simulink model "propulsion_system_simulation_with_solar_powered_battery"  (R2021a)
settings: Solver=VariableStepAuto  StartTime=0.0  StopTime=0.025  FixedStep=0.01  RelTol=1e-3
InitFcn:
  | prop_init_set
undefined symbols (not defined in the file or in its folder): Cp_total, Ct_total
libraries: spspowerguiLib x1
settings Model: SimulationMode=accelerator  Creator=76568  LastModifiedBy=76568

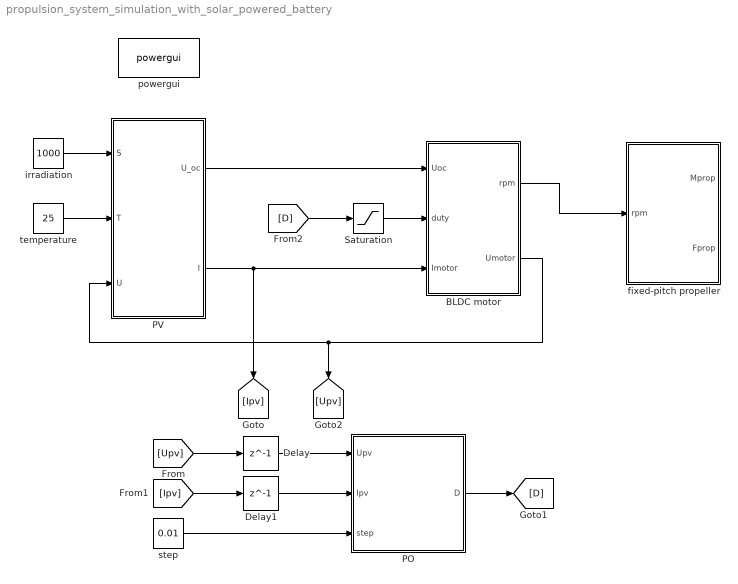
== system propulsion_system_simulation_with_solar_powered_battery ==
  BLDC motor : Subsystem  mask{Kv=125, Rm=0.184}
  Delay : Delay  DelayLength=1
  Delay1 : Delay  DelayLength=1
  PO : MATLAB Function  TreatAsAtomicUnit=on
  PV : Subsystem  mask{Uoc=31.464, Um=26.542, Isc=6.26, Im=5.87}
  Saturation : Saturate  UpperLimit=1  LowerLimit=0
  fixed-pitch propeller : Subsystem  mask{air_speed=10, prop_diameter=0.473, T_static=16.1936, T_max=6.85, V_max=15, air_rho=1.225}
  irradiation : Constant  Value=1000
  powergui : spspowerguiLib/powergui  Priority=1  SimulationMode=Continuous  SampleTime=0.01  frequency=60  Iterations=50  frequencyindice=0  Pbase=100e6  ErrMax=1e-4  UnitsV=kV  UnitsW=MW  buscounter=0  FunctionMessages=off  echomessages=off  EnableUseOfTLC=off  CurrentSourceSwitches=off  DisableSnubberDevices=off  DisableRonSwitches=off  DisableVfSwitches=off  DisplayEquations=off  AutomaticDiscreteSolvers=off  SolverType=Tustin/Backward Euler (TBE)  Interpol=off  ExternalGateDelay=off  methode=off  Ts=100  x0status=blocks  SPID=on  SwTol=0  HookPort=off  NonlinearTolerance=1e-4  nMaxIteration=100  ContinueOnMaxIteration=off  RestoreLinks=warning  ResistiveCurrentMeasurement=off  Frange=[0:2:500]  Ylog=off  Xlog=on  ShowGrid=off  save=off  variable=ZData  structure=0  ZoomFFT=off  StartTime=0.0  cycles=1  DisplayStyle=1  fundamental=60  FreqAxis=off  MaxFrequency=1000  frequencyindicesteady=1  RmsSteady=1  display=off
  step : Constant  Value=0.01
  temperature : Constant  Value=25
  wires:
  [Ipv] -> Delay1/1
  [Upv] -> Delay/1
  step/1 -> PO/3(step)
  PO/1(D) -> [D]
  irradiation/1 -> PV/1(S)
  temperature/1 -> PV/2(T)
  BLDC motor/1(rpm) -> fixed-pitch propeller/1(rpm)
  Saturation/1 -> BLDC motor/2(duty)
  Delay/1 -> PO/1(Upv)
  Delay1/1 -> PO/2(Ipv)
  [D] -> Saturation/1
  PV/1(U_oc) -> BLDC motor/1(Uoc)
  PV/2(I) -> [Ipv], BLDC motor/3(Imotor)
  BLDC motor/2(Umotor) -> [Upv], PV/3(U)

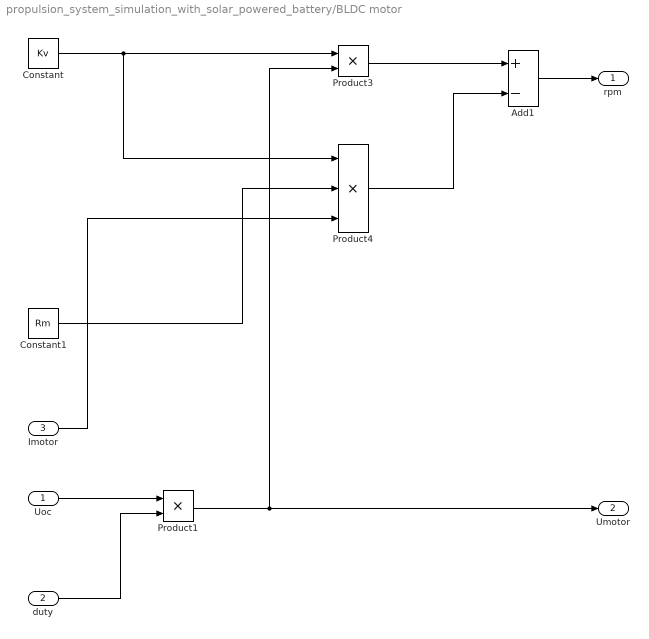
== system propulsion_system_simulation_with_solar_powered_battery/BLDC motor ==
  Uoc : Inport
  duty : Inport  Port=2
  Imotor : Inport  Port=3
  Add1 : Sum  Inputs=+-
  Constant : Constant  Value=Kv
  Constant1 : Constant  Value=Rm
  Product1 : Product
  Product3 : Product  Inputs=**
  Product4 : Product  Inputs=***
  rpm : Outport
  Umotor : Outport  Port=2
  wires:
  Constant/1 -> Product4/1, Product3/1
  Constant1/1 -> Product4/2
  Product3/1 -> Add1/1
  Product4/1 -> Add1/2
  duty/1 -> Product1/2
  Add1/1 -> rpm/1
  Imotor/1 -> Product4/3
  Uoc/1 -> Product1/1
  Product1/1 -> Umotor/1, Product3/2

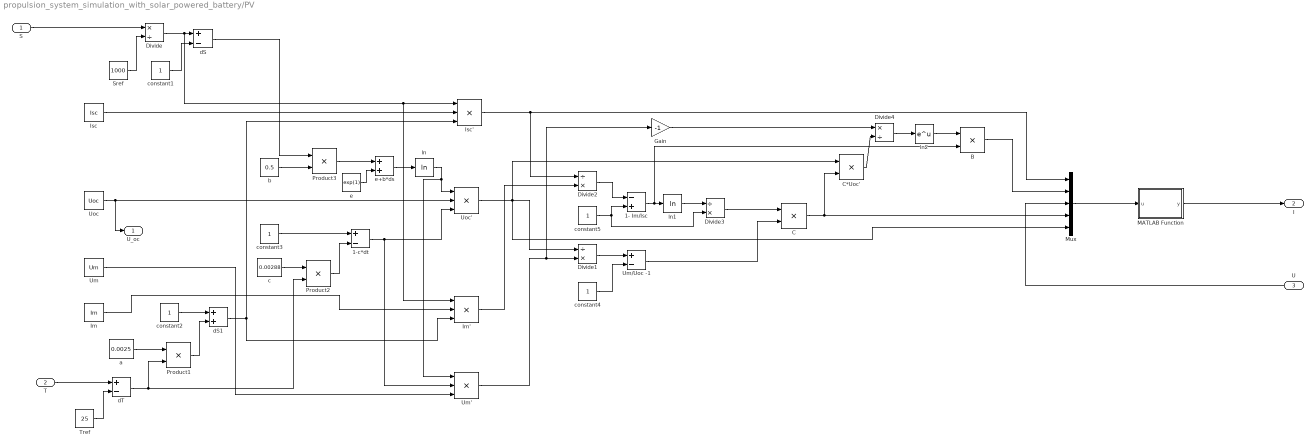
== system propulsion_system_simulation_with_solar_powered_battery/PV ==
  S : Inport
  T : Inport  Port=2
  U : Inport  Port=3
  1- Im/Isc : Sum  Inputs=-+
  1-c*dt : Sum  Inputs=+-
  B : Product
  C : Product
  C*Uoc' : Product
  Divide : Product  Inputs=*/
  Divide1 : Product  Inputs=/*
  Divide2 : Product  Inputs=/*
  Divide3 : Product  Inputs=/*
  Divide4 : Product  Inputs=*/
  Gain : Gain  Gain=-1
  Im : Constant  Value=Im
  Im' : Product  Inputs=3
  Isc : Constant  Value=Isc
  Isc' : Product  Inputs=3
  MATLAB Function : MATLAB Function  TreatAsAtomicUnit=on
  Mux : Mux  Inputs=5
  Product1 : Product
  Product2 : Product
  Product3 : Product
  Sref : Constant  Value=1000
  Tref : Constant  Value=25
  Um : Constant  Value=Um
  Um' : Product  Inputs=3
  Um/Uoc -1 : Sum  Inputs=+-
  Uoc : Constant  Value=Uoc
  Uoc' : Product  Inputs=3
  a : Constant  Value=0.0025
  b : Constant  Value=0.5
  c : Constant  Value=0.00288
  constant{1..5} (5 alike) : Constant
  dS : Sum  Inputs=+-
  dS1 : Sum
  dT : Sum  Inputs=+-
  e : Constant  Value=exp(1)
  e+b*ds : Sum
  ln : Math  Operator=log  SaturateOnIntegerOverflow=on
  ln1 : Math  Operator=log  SaturateOnIntegerOverflow=on
  ln2 : Math  SaturateOnIntegerOverflow=on
  U_oc : Outport
  I : Outport  Port=2
  wires:
  T/1 -> dT/1
  Tref/1 -> dT/2
  S/1 -> Divide/1
  Sref/1 -> Divide/2
  Divide/1 -> Isc'/1, Im'/1, dS/1
  constant1/1 -> dS/2
  a/1 -> Product1/1
  dT/1 -> Product2/2, Product1/2
  constant2/1 -> dS1/1
  Product1/1 -> dS1/2
  dS1/1 -> Im'/3, Isc'/3
  Isc/1 -> Isc'/2
  Uoc/1 -> U_oc/1, Uoc'/2
  constant3/1 -> 1-c*dt/1
  Product2/1 -> 1-c*dt/2
  c/1 -> Product2/1
  1-c*dt/1 -> Um'/2, Uoc'/3
  b/1 -> Product3/2
  dS/1 -> Product3/1
  e/1 -> e+b*ds/2
  Product3/1 -> e+b*ds/1
  e+b*ds/1 -> ln/1
  ln/1 -> Um'/1, Uoc'/1
  Im/1 -> Im'/2
  Um/1 -> Um'/3
  Um'/1 -> Gain/1, Divide1/2
  Divide1/1 -> Um/Uoc -1/1
  constant4/1 -> Um/Uoc -1/2
  Im'/1 -> Divide2/2
  Isc'/1 -> Mux/1, Divide2/1
  Divide2/1 -> 1- Im/Isc/1
  constant5/1 -> Divide3/2, 1- Im/Isc/2
  1- Im/Isc/1 -> B/2, ln1/1
  ln1/1 -> Divide3/1
  Um/Uoc -1/1 -> C/2
  Divide3/1 -> C/1
  C/1 -> Mux/4, C*Uoc'/2
  Gain/1 -> Divide4/1
  C*Uoc'/1 -> Divide4/2
  Divide4/1 -> ln2/1
  ln2/1 -> B/1
  B/1 -> Mux/2
  Uoc'/1 -> Mux/5, Divide1/1, C*Uoc'/1
  Mux/1 -> MATLAB Function/1(u)
  U/1 -> Mux/3
  MATLAB Function/1(y) -> I/1

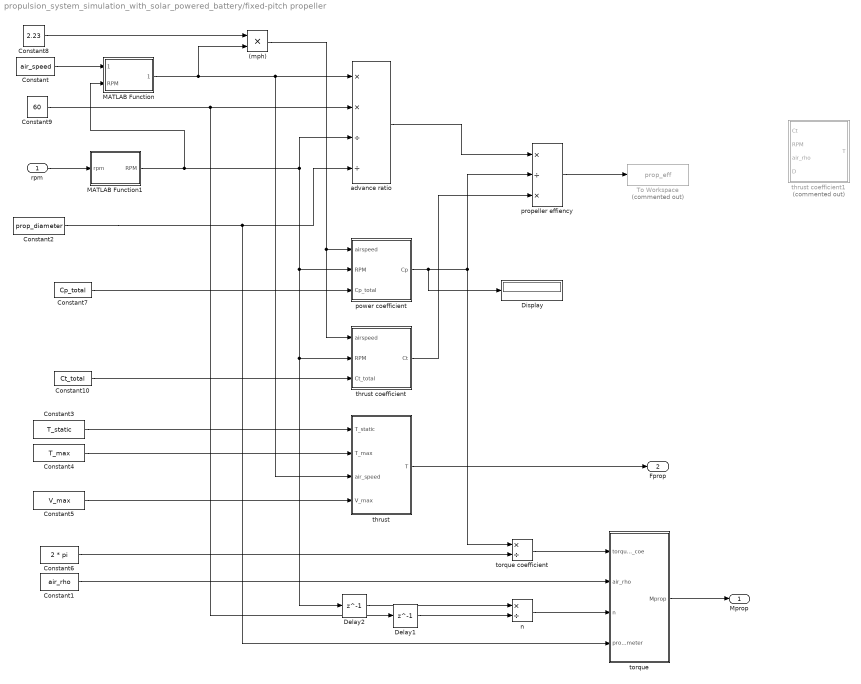
== system propulsion_system_simulation_with_solar_powered_battery/fixed-pitch propeller ==
  rpm : Inport
  (mph) : Product
  Constant : Constant  Value=air_speed
  Constant1 : Constant  Value=air_rho
  Constant10 : Constant  Value=Ct_total
  Constant2 : Constant  Value=prop_diameter
  Constant3 : Constant  Value=T_static
  Constant4 : Constant  Value=T_max
  Constant5 : Constant  Value=V_max
  Constant6 : Constant  Value=2 * pi
  Constant7 : Constant  Value=Cp_total
  Constant8 : Constant  Value=2.23
  Constant9 : Constant  Value=60
  Delay1 : Delay  DelayLength=1  InitialCondition=0  SampleTime=0.0001
  Delay2 : Delay  DelayLength=1  InitialCondition=0  SampleTime=0.0001
  Display : Display
  MATLAB Function : MATLAB Function  TreatAsAtomicUnit=on
  MATLAB Function1 : MATLAB Function  TreatAsAtomicUnit=on
  To Workspace : ToWorkspace  Commented=on  VariableName=prop_eff  SaveFormat=Timeseries  SampleTime=-1
  advance ratio : Product  Inputs=**//
  n : Product  Inputs=*/
  power coefficient : MATLAB Function  TreatAsAtomicUnit=on
  propeller effiency : Product  Inputs=*/*
  thrust : MATLAB Function  TreatAsAtomicUnit=on
  thrust coefficient : MATLAB Function  TreatAsAtomicUnit=on
  thrust coefficient1 : MATLAB Function  Commented=on  TreatAsAtomicUnit=on
  torque : MATLAB Function  TreatAsAtomicUnit=on
  torque coefficient : Product  Inputs=*/
  Mprop : Outport
  Fprop : Outport  Port=2
  wires:
  thrust coefficient/1(Ct) -> propeller effiency/3
  MATLAB Function1/1(RPM) -> MATLAB Function/2(RPM), Delay2/1, thrust coefficient/2(RPM), power coefficient/2(RPM), advance ratio/3
  Constant2/1 -> advance ratio/4, torque/4(prop_diameter)
  advance ratio/1 -> propeller effiency/1
  torque coefficient/1 -> torque/1(torque_coe)
  Constant1/1 -> torque/2(air_rho)
  Constant10/1 -> thrust coefficient/3(Ct_total)
  MATLAB Function/1(airspeed) -> thrust/3(air_speed), advance ratio/1, (mph)/2
  Constant/1 -> MATLAB Function/1(air_speed)
  (mph)/1 -> thrust coefficient/1(airspeed), power coefficient/1(airspeed)
  Constant6/1 -> torque coefficient/2
  n/1 -> torque/3(n)
  Constant8/1 -> (mph)/1
  Constant7/1 -> power coefficient/3(Cp_total)
  Constant9/1 -> Delay1/1, advance ratio/2
  Constant3/1 -> thrust/1(T_static)
  rpm/1 -> MATLAB Function1/1(rpm)
  thrust/1(T) -> Fprop/1
  Constant5/1 -> thrust/4(V_max)
  propeller effiency/1 -> To Workspace/1
  Constant4/1 -> thrust/2(T_max)
  torque/1(Mprop) -> Mprop/1
  power coefficient/1(Cp) -> Display/1, torque coefficient/1, propeller effiency/2
  Delay1/1 -> n/2
  Delay2/1 -> n/1

== matlab function propulsion_system_simulation_with_solar_powered_battery/PV/MATLAB Function ==
  data: u input; y output
function y = fcn(u)
y=u(1)*(1-u(2)*(exp(u(3)/u(4)/u(5))-1));

== matlab function propulsion_system_simulation_with_solar_powered_battery/PO ==
  data: Upv input; D output; Ipv input; step input
function D = MPPT(Upv, Ipv, step)

persistent Prev Urev Drev

if isempty(Prev)
    Drev = 0.5;
    Urev = 0;
    Prev = 0;
end

P = Upv * Ipv;
dP = P - Prev;
dU = Upv - Urev;

if P ~= 0
    if dP > 0
        if dU > 0
            D = Drev + step;
        else
            D = Drev - step;
        end
    else
        if dU > 0
            D = Drev - step;
        else
            D = Drev + step;
        end
    end
else
    D = Drev;
end

Drev = D;
Prev = P;
Urev = Upv;
end

== matlab function propulsion_system_simulation_with_solar_powered_battery/fixed-pitch propeller/power coefficient ==
  data: airspeed input; Cp output; RPM input; Cp_total input
function Cp = fcn(airspeed, RPM, Cp_total)
Cp_temp = interp2(0 : 0.5 : 50, 1000 : 1000 : 5000, Cp_total, airspeed, RPM);
Cp_temp(isnan(Cp_temp)) = 0;
Cp = Cp_temp;

== matlab function propulsion_system_simulation_with_solar_powered_battery/fixed-pitch propeller/thrust ==
  data: T_static input; T output; T_max input; air_speed input; V_max input
function T = fcn(T_static, T_max, air_speed, V_max)
T = ((T_static - 2 * T_max) / V_max ^ 2) * air_speed ^ 2 + ((3 * T_max - 2 * T_static) / V_max) * air_speed + T_static;

== matlab function propulsion_system_simulation_with_solar_powered_battery/fixed-pitch propeller/thrust coefficient ==
  data: airspeed input; Ct output; RPM input; Ct_total input
function Ct = fcn(airspeed, RPM, Ct_total)
Ct_temp = interp2(0 : 0.5 : 50, 1000 : 1000 : 5000, Ct_total, airspeed, RPM);
Ct_temp(isnan(Ct_temp)) = 0;
Ct = Ct_temp;

== matlab function propulsion_system_simulation_with_solar_powered_battery/fixed-pitch propeller/torque ==
  data: torque_coe input; Mprop output; air_rho input; n input; prop_diameter input
function Mprop = fcn(torque_coe, air_rho, n, prop_diameter)
Mprop = torque_coe * air_rho * n ^ 2 * prop_diameter ^ 5;

== matlab function propulsion_system_simulation_with_solar_powered_battery/fixed-pitch propeller/thrust coefficient1 ==
  data: Ct input; T output; RPM input; air_rho input; D input
function T = fcn(Ct, RPM, air_rho, D)
T = air_rho * RPM ^ 2 * D ^ 4 * Ct * 3600;

== matlab function propulsion_system_simulation_with_solar_powered_battery/fixed-pitch propeller/MATLAB Function ==
  data: air_speed input; airspeed output; RPM input
function airspeed = fcn(air_speed, RPM)
if RPM <= 2000
    if air_speed > 8.94
       airspeed = 8.94;
    else
        airspeed = air_speed;
    end
end
if 2000 < RPM <= 3000
    if air_speed > 13.41
        airspeed = 13.41;
    else
        airspeed = air_speed;
    end
end
if 3000 < RPM <= 4000
    if air_speed > 17.88
        airspeed = 17.88;
    else
        airspeed = air_speed;
    end
end
if 4000 < RPM <= 5000
    if air_speed > 22.35
        airspeed = 22.35;
    else
        airspeed = air_speed;
    end
else
    airspeed = air_speed;
end
end

== matlab function propulsion_system_simulation_with_solar_powered_battery/fixed-pitch propeller/MATLAB Function1 ==
  data: rpm input; RPM output
function RPM = fcn(rpm)
if rpm < 1000
    rpm = 1000;
end
if rpm > 5000
    rpm = 5000;
end
RPM = rpm;
end
